simulink model "schemat_transmitancje"  (R2015a)
settings: Solver=ode45  StartTime=0.0  StopTime=4000  MaxStep=400  RelTol=1e-3
values from neighbouring files (symbols this model uses):
  A = [cpf*Cvp cpf*(Kp+K2)]    [mini_projekt_6b_baza.m]    (also in symulacje_bez_simulinka.m = [-(cpf + K1 + Kp)/Cvw, Kp/Cvw; Kp/Cvp, -(Kp+K2)/Cvp])
  B = [K1*Cvp K1*(Kp+K2)+(Kp*K2)]    [mini_projekt_6b_baza.m]    (also in symulacje_bez_simulinka.m = [cpf/Cvw, K1/Cvw;0,  K2/Cvp])
  C = [cpf*Kp]    [mini_projekt_6b_baza.m]    (also in symulacje_bez_simulinka.m = [1, 0; 0, 1])
  D = [(K2*Cvw) K2*(cpf+K1+Kp)+(Kp*K1)]    [mini_projekt_6b_baza.m]    (also in symulacje_bez_simulinka.m = [0, 0; 0, 0])
  dTkz = 0    [mini_projekt_6b_baza.m]    (also in symulacje_bez_simulinka.m = 2)
  dTzew = 0    [mini_projekt_6b_baza.m]    (also in symulacje_bez_simulinka.m = 2)
  M = [(Cvw*Cvp) (Cvp*(cpf+K1+Kp) + Cvw*(Kp+K2)) ((Kp+K2)*(cpf+K1+Kp)-Kp^2)]    [mini_projekt_6b_baza.m]    (also in symulacje_bez_simulinka.m = 1/(K2+Kp))
  t0 = 5000    [mini_projekt_6b_baza.m]    (also in symulacje_bez_simulinka.m)
  Tpo1 = M*(Kp*Twewo1+K2*Tzewo)    [mini_projekt_6b_baza.m]
  Twewo1 = (cpf*Tkzo+K1*Tzewo+Kp*K2*M*Tzewo)/(cpf+K1+Kp-M*Kp^2)    [mini_projekt_6b_baza.m]
settings Model: Creator=hoacy_000  LastModifiedBy=apuch
settings DebuggingCC: UnderspecifiedInitializationDetection=Classic  MergeDetectMultiDrivingBlocksExec=none  SolverPrmCheckMsg=warning

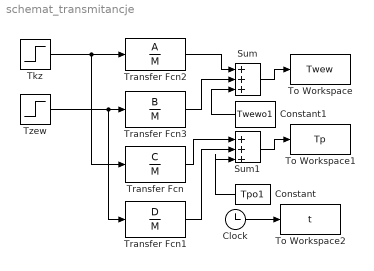
== system schemat_transmitancje ==
  Clock : Clock
  Constant : Constant  Value=Tpo1
  Constant1 : Constant  Value=Twewo1
  Sum : Sum  Inputs=+++
  Sum1 : Sum  Inputs=|+++
  Tkz : Step  Time=t0  After=0+dTkz  SampleTime=0
  To Workspace : ToWorkspace  VariableName=Twew  SampleTime=-1
  To Workspace1 : ToWorkspace  VariableName=Tp  SampleTime=-1
  To Workspace2 : ToWorkspace  VariableName=t  SampleTime=-1
  Transfer Fcn : TransferFcn  Numerator=C  Denominator=M
  Transfer Fcn1 : TransferFcn  Numerator=D  Denominator=M
  Transfer Fcn2 : TransferFcn  Numerator=A  Denominator=M
  Transfer Fcn3 : TransferFcn  Numerator=B  Denominator=M
  Tzew : Step  Time=t0  After=0+dTzew  SampleTime=0
  wires:
  Sum/1 -> To Workspace/1
  Sum1/1 -> To Workspace1/1
  Tkz/1 -> Transfer Fcn/1, Transfer Fcn2/1
  Tzew/1 -> Transfer Fcn1/1, Transfer Fcn3/1
  Transfer Fcn2/1 -> Sum/1
  Transfer Fcn3/1 -> Sum/2
  Transfer Fcn/1 -> Sum1/1
  Transfer Fcn1/1 -> Sum1/2
  Clock/1 -> To Workspace2/1
  Constant/1 -> Sum1/3
  Constant1/1 -> Sum/3
